simulink model "StoreSimulation"  (R2024b)
settings: Solver=VariableStepAuto  StartTime=0.0  StopTime=10.0  RelTol=1e-3
settings Model: Creator=CArias  LastModifiedBy=CArias

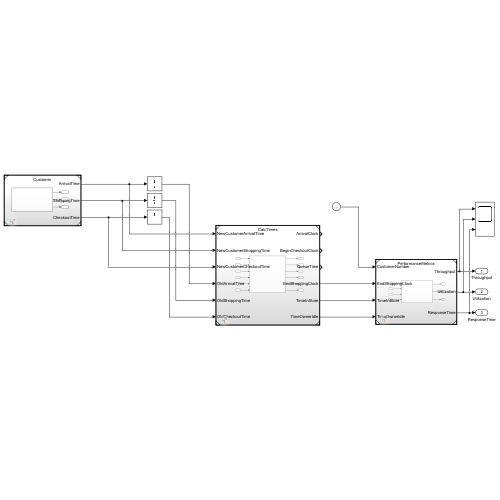
[thumbnail: Simulink's stored preview of the top-level diagram]
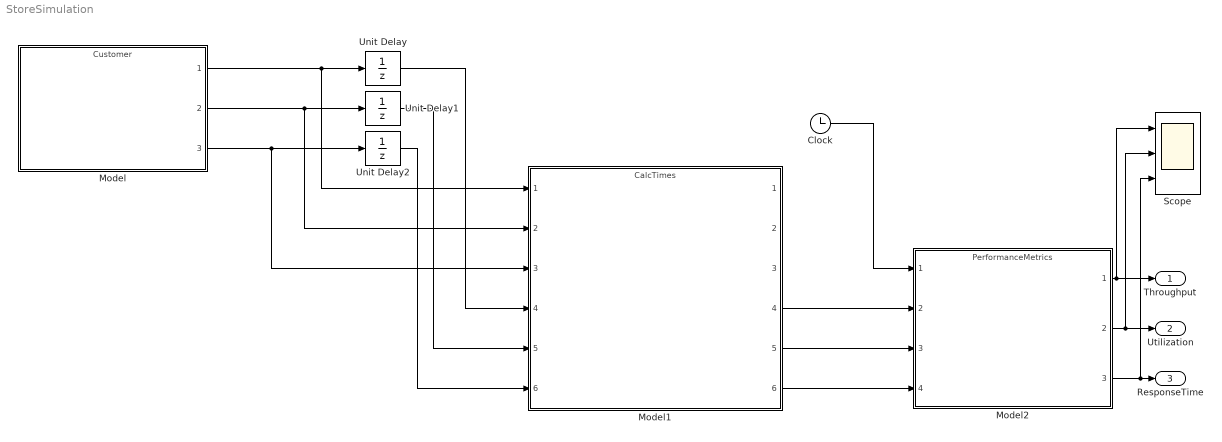
== system StoreSimulation ==
  Clock : Clock
  Model : ModelReference  ModelNameDialog=Customer.slx  SimulationMode=Normal  ModelReferenceVersion=1.1
  Model1 : ModelReference  ModelNameDialog=CalcTimes.slx  SimulationMode=Normal  ModelReferenceVersion=1.5
  Model2 : ModelReference  ModelNameDialog=PerformanceMetrics.slx  SimulationMode=Normal  ModelReferenceVersion=1.2
  Scope : Scope  NumInputPorts=3
  Unit Delay : UnitDelay  SampleTime=-1  HasFrameUpgradeWarning=on
  Unit Delay1 : UnitDelay  SampleTime=-1  HasFrameUpgradeWarning=on
  Unit Delay2 : UnitDelay  SampleTime=-1  HasFrameUpgradeWarning=on
  Throughput : Outport
  Utilization : Outport  Port=2
  ResponseTime : Outport  Port=3
  wires:
  Model/1 -> Unit Delay/1, Model1/1
  Model/2 -> Unit Delay1/1, Model1/2
  Model/3 -> Unit Delay2/1, Model1/3
  Unit Delay/1 -> Model1/4
  Unit Delay1/1 -> Model1/5
  Unit Delay2/1 -> Model1/6
  Model1/5 -> Model2/3
  Model1/4 -> Model2/2
  Model1/6 -> Model2/4
  Clock/1 -> Model2/1
  Model2/1 -> Throughput/1, Scope/1
  Model2/2 -> Utilization/1, Scope/2
  Model2/3 -> Scope/3, ResponseTime/1
